simulink model "weight_transfer"  (R2024b)
settings: Solver=VariableStepAuto  StartTime=0.0  StopTime=10.0  RelTol=1e-3
libraries: simulink_extras x5, vehdynlibsteering x1
settings Model: Creator=beras  LastModifiedBy=beras

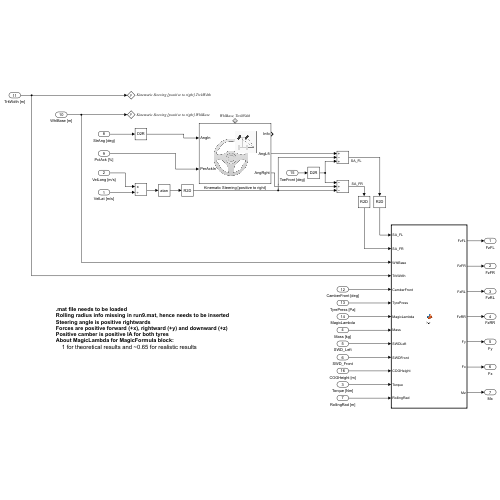
[thumbnail: Simulink's stored preview of the top-level diagram]
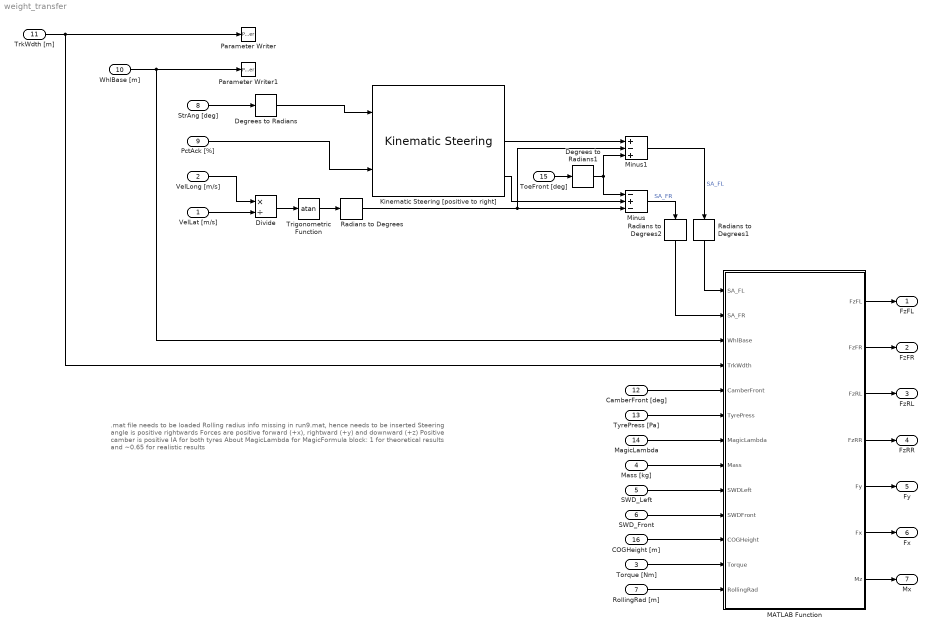
== system weight_transfer ==
  note: .mat file needs to be loaded
      | Rolling radius info missing in run9.mat, hence needs to be inserted
      | Steering angle is positive rightwards
      | Forces are positive forward (+x), rightward (+y) and downward (+z)
      | Positive camber is positive IA for both tyres
      | About MagicLambda for MagicFormula block:
      | 1 for theoretical results and ~0.65 for realistic results
  VelLat [m/s] : Inport
  VelLong [m/s] : Inport  Port=2
  Torque [Nm] : Inport  Port=3
  Mass [kg] : Inport  Port=4
  SWD_Left : Inport  Port=5
  SWD_Front : Inport  Port=6
  RollingRad [m] : Inport  Port=7
  StrAng [deg] : Inport  Port=8
  PctAck [%] : Inport  Port=9
  WhlBase [m] : Inport  Port=10
  TrkWdth [m] : Inport  Port=11
  CamberFront [deg] : Inport  Port=12
  TyrePress [Pa] : Inport  Port=13
  MagicLambda : Inport  Port=14
  ToeFront [deg] : Inport  Port=15
  COGHeight [m] : Inport  Port=16
  Degrees to Radians : simulink_extras/Transformations/Degrees to Radians
  Degrees to Radians1 : simulink_extras/Transformations/Degrees to Radians
  Divide : Product  Inputs=*/
  Kinematic Steering [positive to right] : vehdynlibsteering/Kinematic Steering  StrgType=Ackerman  StrgRatioType=Constant  Loc=Front  NrmlFctr=1  TrckWdth=1  WhlBase=1  Db=0  StrgRng=1.25*pi  StrgAngBpts="[-6.2832   -5.0265   -3.7699   -2.5133   -1.2566         0    1.2566    2.5133    3.7699    5.0265    6.2832]"  StrgRatioTbl=|  StrgRatio=100  PctAckIn=on  PctAck=100  PctAckTbl=ones(1,11)*100  StrgArmLngth=0.1  RckCsLngth=0.5  TieRodLngth=0.248  D=0.2  PnnRadius=0.00085818  PnnRadiusTbl="[0.0055    0.0055    0.0056    0.0057    0.0058    0.0057    0.0057    0.0057    0.0056    0.0055    0.0055]"  RodLngth=0.1  ParaArmLngth=0.9  aMode=2
      | [13.5000   13.3750   13.2500   13.1250   13.0000   13.0000   13.0000   13.1250   13.2500   13.3750   13.5000
      | ]
  MATLAB Function : MATLAB Function  TreatAsAtomicUnit=on
  Minus : Sum  Inputs=-+-
  Minus1 : Sum  Inputs=+-+
  Parameter Writer : ParameterWriter  ParameterOwnerBlock=../Kinematic Steering [positive to right]  ParameterName=TrckWdth  ParameterInternalName=TrckWdth
  Parameter Writer1 : ParameterWriter  ParameterOwnerBlock=../Kinematic Steering [positive to right]  ParameterName=WhlBase  ParameterInternalName=WhlBase
  Radians to Degrees : simulink_extras/Transformations/Radians to Degrees
  Radians to Degrees1 : simulink_extras/Transformations/Radians to Degrees
  Radians to Degrees2 : simulink_extras/Transformations/Radians to Degrees
  Trigonometric Function : Trigonometry  Operator=atan
  FzFL : Outport
  FzFR : Outport  Port=2
  FzRL : Outport  Port=3
  FzRR : Outport  Port=4
  Fy : Outport  Port=5
  Fx : Outport  Port=6
  Mx : Outport  Port=7
  wires:
  VelLong [m/s]/1 -> Divide/1
  VelLat [m/s]/1 -> Divide/2
  Divide/1 -> Trigonometric Function/1
  Trigonometric Function/1 -> Radians to Degrees/1
  StrAng [deg]/1 -> Degrees to Radians/1
  PctAck [%]/1 -> Kinematic Steering [positive to right]/2
  WhlBase [m]/1 -> MATLAB Function/3(WhlBase), Parameter Writer1/1
  TrkWdth [m]/1 -> MATLAB Function/4(TrkWdth), Parameter Writer/1
  Kinematic Steering [positive to right]/2 -> Minus1/1
  Kinematic Steering [positive to right]/3 -> Minus/2
  Degrees to Radians/1 -> Kinematic Steering [positive to right]/1
  ToeFront [deg]/1 -> Degrees to Radians1/1
  Minus1/1 -> Radians to Degrees1/1  "SA_FL"
  Minus/1 -> Radians to Degrees2/1  "SA_FR"
  Radians to Degrees/1 -> Minus/3, Minus1/2
  Degrees to Radians1/1 -> Minus/1, Minus1/3
  CamberFront [deg]/1 -> MATLAB Function/5(CamberFront)
  TyrePress [Pa]/1 -> MATLAB Function/6(TyrePress)
  MagicLambda/1 -> MATLAB Function/7(MagicLambda)
  Mass [kg]/1 -> MATLAB Function/8(Mass)
  SWD_Left/1 -> MATLAB Function/9(SWDLeft)
  SWD_Front/1 -> MATLAB Function/10(SWDFront)
  COGHeight [m]/1 -> MATLAB Function/11(COGHeight)
  Torque [Nm]/1 -> MATLAB Function/12(Torque)
  RollingRad [m]/1 -> MATLAB Function/13(RollingRad)
  MATLAB Function/4(FzRR) -> FzRR/1
  MATLAB Function/3(FzRL) -> FzRL/1
  MATLAB Function/2(FzFR) -> FzFR/1
  MATLAB Function/1(FzFL) -> FzFL/1
  Radians to Degrees2/1 -> MATLAB Function/2(SA_FR)
  Radians to Degrees1/1 -> MATLAB Function/1(SA_FL)
  MATLAB Function/6(Fx) -> Fx/1
  MATLAB Function/7(Mz) -> Mx/1
  MATLAB Function/5(Fy) -> Fy/1

== matlab function weight_transfer/MATLAB Function ==
  data: SA_FL input; SA_FR input; WhlBase input; TrkWdth input; FzFL output; FzFR output; FzRL output; FzRR output; CamberFront input; TyrePress input; MagicLambda input; Mass input; SWDLeft input; SWDFront input; COGHeight input; Torque input; RollingRad input; Fy output; Fx output; Mz output
function [FzFL,FzFR,FzRL,FzRR,Fy,Fx,Mz] = fcn(SA_FL,SA_FR,WhlBase,TrkWdth,...
    CamberFront,TyrePress,MagicLambda,Mass,SWDLeft,SWDFront,COGHeight,...
    Torque,RollingRad)

% Forces are positive forward (+x), rightward (+y) and downward (+z)
%
%    Tyre testing convention:
% - Turning left is positive SA for both tyres
% - Positive camber is positive IA for the right tyre
% - Positive camber is negative IA for the left tyre
%
%    Due to assymetric Fy vs SA response, the convention is flipped for
%    the left tyre:
% - Positive camber is positive IA for both tyres
% - Turning left is negative SA for the left tyre
% - Turning left is positive SA for the right tyre (unchanged)
%
% Furthermore, the Ackermann steering block gives positive SA for
% turning right, hence
SA_FR=-SA_FR;
% Fy_FR hence will also need to be reversed


mfparams.UNLOADED_RADIUS=RollingRad; % filling missing data
weight=Mass*9.81;
Press=TyrePress;
MagicLambda=MagicLambda;

% Initialisation with static weight distribution
Fz_FL_static=weight*SWDFront*SWDLeft;
Fz_FR_static=weight*SWDFront*(1-SWDLeft);
Fz_RL_static=weight*(1-SWDFront)*SWDLeft;
Fz_RR_static=weight*(1-SWDFront)*(1-SWDLeft);
Fz_FL_new=Fz_FL_static;
Fz_FR_new=Fz_FR_static;
Fz_RL_new=Fz_RL_static;
Fz_RR_new=Fz_RR_static;

% Rear COF
SA=0;
Fz=min(Fz_RL_new,Fz_RR_new);
IA=0;
RearMagic=sim('MagicFormula_matlab');
COFRear=getdatasamples(RearMagic.mu_y,1)*MagicLambda; % Questionable

% Placeholder values for while loop
Fz_FL_old=2*Fz_FL_new;
Fz_FR_old=2*Fz_FR_new;
Fz_RL_old=2*Fz_RL_new;
Fz_RR_old=2*Fz_RR_new;

% Rolling ignored for now
IA=CamberFront;

epsilon=0.01; % Acceptable error (kind of)
% Iterate while the change between iterations in any corner is larger
% than epsilon
while abs(1-Fz_FL_old/Fz_FL_new)>epsilon ||...
        abs(1-Fz_FR_old/Fz_FR_new)>epsilon ||...
        abs(1-Fz_RL_old/Fz_RL_new)>epsilon ||...
        abs(1-Fz_RR_old/Fz_RR_new)>epsilon

    SA=SA_FL;
    Fz=Fz_FL_new;
    FL=sim('MagicFormula_matlab');
    Fy_FL=-getdatasamples(FL.Fy,1);
    % negative due to different coordinate systems (i think?)

    SA=SA_FR;
    Fz=Fz_FR_new;
    FR=sim('MagicFormula_matlab');
    Fy_FR=getdatasamples(FR.Fy,1);
    % as mentioned needs to be reversed, hence double negative

    if abs(Fy_FL)>abs(Fy_FR)
        Fy=2*Fy_FR;
    else
        Fy=2*Fy_FL;
    end

    ay=Fy/(mass*9.81); % in g's

    Fx_max=min(Fz_RL_new,Fz_RR_new)*COFRear*RollingRad;
    if Torque==0
        Fx=0;
    elseif abs(Torque)<Fx_max
        Fx=2*Torque/RollingRad;
    else
        if Torque<0
            Fx=-2*Fx_max;
        else
            Fx=2*Fx_max;
        end
    end

    ax=Fx/(mass*9.81); % in g's

    LatTrans=weight*ay*COGHeight/TrkWdth;
    LongTrans=weight*ax*COGHeight/WhlBase;

    Fz_FL_old=Fz_FL_new;
    Fz_FR_old=Fz_FR_new;
    Fz_RL_old=Fz_RL_new;
    Fz_RR_old=Fz_RR_new;

    Fz_FL_new=Fz_FL_static+LatTrans-LongTrans;
    Fz_FR_new=Fz_FR_static-LatTrans-LongTrans;
    Fz_RL_new=Fz_RL_static+LatTrans+LongTrans;
    Fz_RR_new=Fz_RR_static-LatTrans+LongTrans;
end

Mz_FL=-getdatasamples(FL.Mz,1);
Mz_FR=getdatasamples(FR.Mz,1);

if abs(Mz_FL)>abs(Mz_FR) % Like with Fy and Fx, the smaller Mz is assumed
    Mz=Mz_FR;
else
    Mz=Mz_FL;
end


FzFL=Fz_FL_new;
FzFR=Fz_FR_new;
FzRL=Fz_FL_new;
FzRR=Fz_FR_new;
